simulink model "Simulink10"  (R2016b)
settings: Solver=VariableStepAuto  StartTime=0.0  StopTime=50  RelTol=1e-3
values from neighbouring files (symbols this model uses):
  A = [0 0 1 0 0 0 ... (first row only)    [Ejercicio10.m]
  B = [0 0 ... (first row only)    [Ejercicio10.m]
  C = [1 0 0 0 0 0 ... (first row only)    [Ejercicio10.m]
  D = zeros(2,2)    [Ejercicio10.m]
  Kc = lqr(A,B,Q,R)    [Ejercicio10.m]
  Kff = [m_heli*g*l_cm/Kpp; 0]    [Ejercicio10.m]
  VMAX_AMP = [24; 15]    [Ejercicio10.m]
settings Model: Creator=mluser  LastModifiedBy=elena
settings DataIOCC: ReturnWorkspaceOutputs=on
settings DebuggingCC: SFMachineParentedDataDiag=error
settings SFSimCC: SimUseLocalCustomCode=on
settings RTWCC: RTWUseLocalCustomCode=on

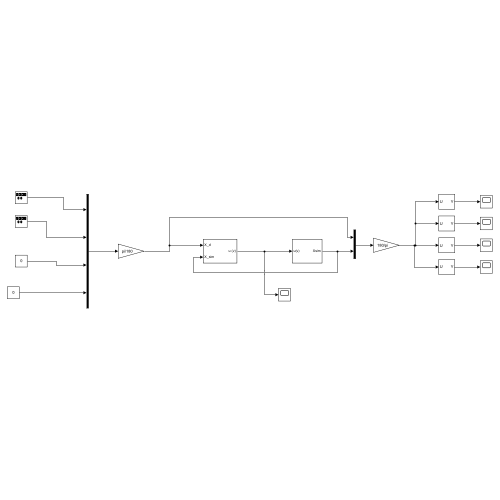
[thumbnail: Simulink's stored preview of the top-level diagram]
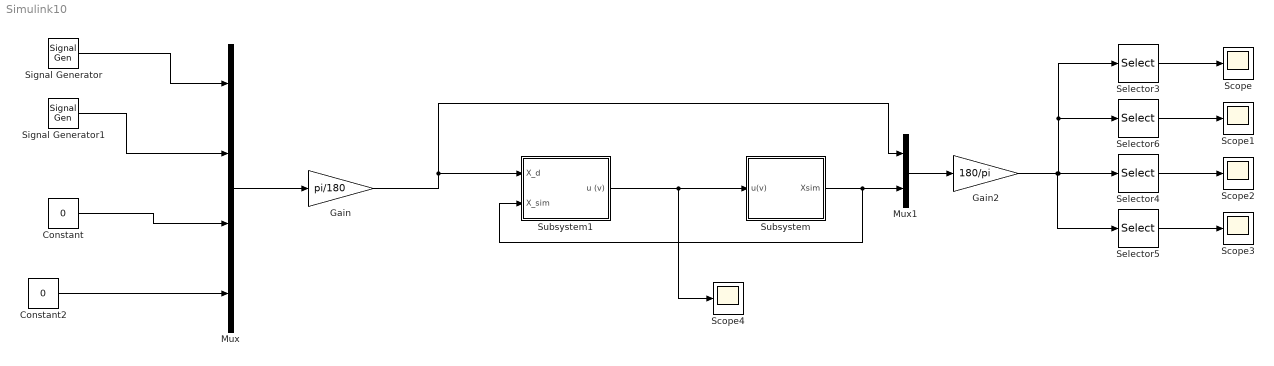
== system Simulink10 ==
  Constant : Constant  Value=0
  Constant2 : Constant  Value=0
  Gain : Gain  Gain=pi/180
  Gain2 : Gain  Gain=180/pi
  Mux : Mux
  Mux1 : Mux  Inputs=2
  Scope{,1..4} (5 alike) : Scope
  Selector3 : Selector  InputPortWidth=8  IndexOptions=Index vector (dialog)  Indices=[1 5]  OutputSizes=1
  Selector4 : Selector  InputPortWidth=8  IndexOptions=Index vector (dialog)  Indices=[3 7]  OutputSizes=1
  Selector5 : Selector  InputPortWidth=8  IndexOptions=Index vector (dialog)  Indices=[4 8]  OutputSizes=1
  Selector6 : Selector  InputPortWidth=8  IndexOptions=Index vector (dialog)  Indices=[2 6]  OutputSizes=1
  Signal Generator : SignalGenerator  WaveForm=square  Amplitude=10  Frequency=0.05
  Signal Generator1 : SignalGenerator  WaveForm=square  Frequency=0.05
  Subsystem : Subsystem
  Subsystem1 : Subsystem
  wires:
  Signal Generator/1 -> Mux/1
  Signal Generator1/1 -> Mux/2
  Mux/1 -> Gain/1
  Gain/1 -> Subsystem1/1(X_d), Mux1/1
  Subsystem/1(Xsim) -> Subsystem1/2(X_sim), Mux1/2
  Mux1/1 -> Gain2/1
  Gain2/1 -> Selector5/1, Selector4/1, Selector6/1, Selector3/1
  Constant/1 -> Mux/3
  Constant2/1 -> Mux/4
  Subsystem1/1(u (v)) -> Scope4/1, Subsystem/1(u(v))
  Selector3/1 -> Scope/1
  Selector6/1 -> Scope1/1
  Selector4/1 -> Scope2/1
  Selector5/1 -> Scope3/1

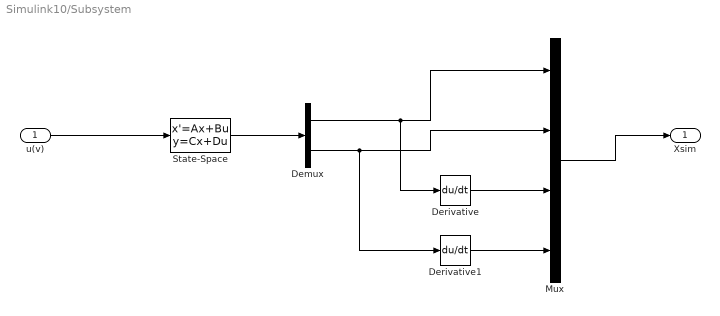
== system Simulink10/Subsystem ==
  u(v) : Inport
  Demux : Demux  Outputs=2
  Derivative : Derivative
  Derivative1 : Derivative
  Mux : Mux
  State-Space : StateSpace  A=A  B=B  C=C  D=D  X0=0
  Xsim : Outport
  wires:
  u(v)/1 -> State-Space/1
  State-Space/1 -> Demux/1
  Mux/1 -> Xsim/1
  Demux/1 -> Derivative/1, Mux/1
  Demux/2 -> Derivative1/1, Mux/2
  Derivative/1 -> Mux/3
  Derivative1/1 -> Mux/4

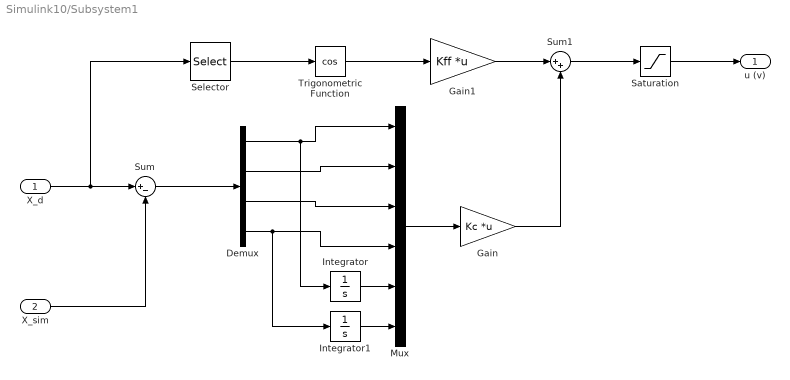
== system Simulink10/Subsystem1 ==
  X_d : Inport
  X_sim : Inport  Port=2
  Demux : Demux
  Gain : Gain  Gain=Kc  Multiplication=Matrix(K*u)
  Gain1 : Gain  Gain=Kff  Multiplication=Matrix(K*u)
  Integrator : Integrator
  Integrator1 : Integrator
  Mux : Mux  Inputs=6
  Saturation : Saturate  UpperLimit=VMAX_AMP  LowerLimit=-VMAX_AMP
  Selector : Selector  InputPortWidth=4  IndexOptions=Index vector (dialog)  Indices=[1]  OutputSizes=1
  Sum : Sum  Inputs=|+-
  Sum1 : Sum  Inputs=|++
  Trigonometric Function : Trigonometry  Operator=cos
  u (v) : Outport
  wires:
  X_d/1 -> Selector/1, Sum/1
  X_sim/1 -> Sum/2
  Sum/1 -> Demux/1
  Demux/1 -> Integrator/1, Mux/1
  Demux/2 -> Mux/2
  Demux/3 -> Mux/3
  Demux/4 -> Integrator1/1, Mux/4
  Integrator/1 -> Mux/5
  Integrator1/1 -> Mux/6
  Mux/1 -> Gain/1
  Selector/1 -> Trigonometric Function/1
  Trigonometric Function/1 -> Gain1/1
  Gain1/1 -> Sum1/1
  Gain/1 -> Sum1/2
  Saturation/1 -> u (v)/1
  Sum1/1 -> Saturation/1
